simulink model "SalientPolePMSM"  (R2020b)
settings: Solver=VariableStepAuto  StartTime=0  StopTime=1  MaxStep=1e-4  RelTol=1e-4
values from neighbouring files (symbols this model uses):
  Bgain = 1    [DataSalientPolePMSM-DESKTOP-IINSHMA.m]    (also in DataSalientPolePMSM.m)
  Gcc_1ord = 1/(s/bandwidth(Gcc) + 1)    [DataSalientPolePMSM-DESKTOP-IINSHMA.m]    (also in DataSalientPolePMSM.m)
  lamdVec = mot.Ld*idVec+mot.lammg    [DataSalientPolePMSM-DESKTOP-IINSHMA.m]    (also in DataSalientPolePMSM.m)
  lamqVec = mot.Lq*iqVec    [DataSalientPolePMSM-DESKTOP-IINSHMA.m]    (also in DataSalientPolePMSM.m)
  TAB0_abc = Tabc_AB0^-1    [DataSalientPolePMSM-DESKTOP-IINSHMA.m]    (also in DataSalientPolePMSM.m)
  Tabc_AB0 = 2/3.*[     1       -1/2       -1/2 ... (first row only)    [DataSalientPolePMSM-DESKTOP-IINSHMA.m]    (also in DataSalientPolePMSM.m)
  Talphabeta_abc = Tabc_alphabeta^(-1)    [DataSalientPolePMSM-DESKTOP-IINSHMA.m]    (also in DataSalientPolePMSM.m)
undefined symbols (not defined in the file or in its folder): DiscIntNeverNeededParam, dqpll, inv, kid, kpd, magnitude, meas, mot, Obs, PI, stconv
libraries: simulink x53, pid_lib x3, powerlib x2, eeBldcCommutationLogic x1, electricdrivelib x1
(part 5 of 7)

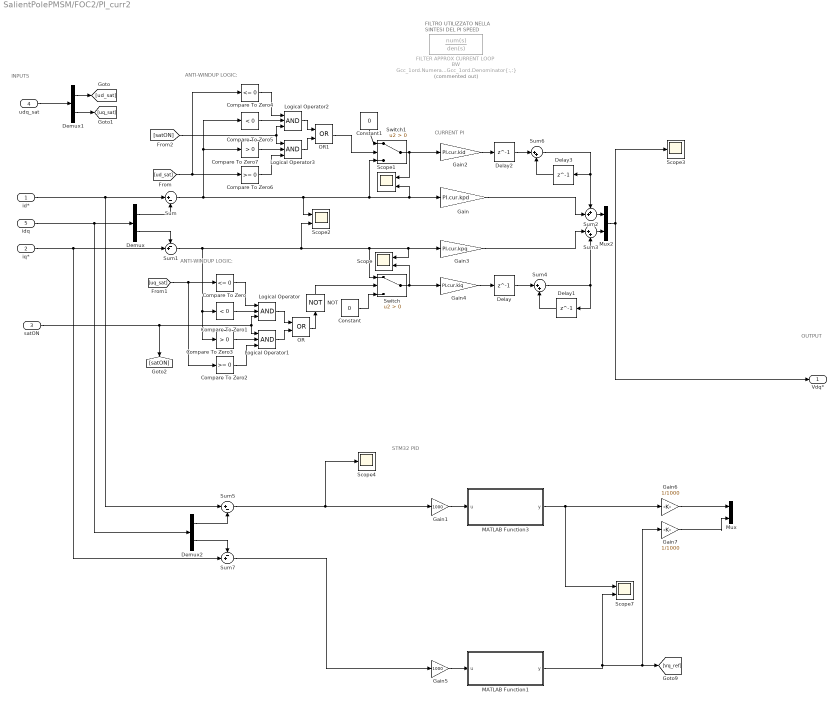
== system SalientPolePMSM/FOC2/PI_curr2 ==
  note: INPUTS
  note: OUTPUT
  note: ANTI-WINDUP LOGIC:
  note: ANTI-WINDUP LOGIC:
  note: STM32 PID
  note: FILTRO UTILIZZATO
      | NELLA SINTESI DEL
      | PI SPEED
  note: CURRENT PI
  id* : Inport
  iq* : Inport  Port=2
  satON : Inport  Port=3
  udq_sat : Inport  Port=4
  idq : Inport  Port=5
  Compare To Zero : simulink/Logic and Bit Operations/Compare To Zero  relop=<=  OutDataTypeStr=boolean  ZeroCross=off
  Compare To Zero1 : simulink/Logic and Bit Operations/Compare To Zero  relop=<  OutDataTypeStr=boolean  ZeroCross=off
  Compare To Zero2 : simulink/Logic and Bit Operations/Compare To Zero  relop=>=  OutDataTypeStr=boolean  ZeroCross=off
  Compare To Zero3 : simulink/Logic and Bit Operations/Compare To Zero  relop=>  OutDataTypeStr=boolean  ZeroCross=off
  Compare To Zero4 : simulink/Logic and Bit Operations/Compare To Zero  relop=<=  OutDataTypeStr=boolean  ZeroCross=off
  Compare To Zero5 : simulink/Logic and Bit Operations/Compare To Zero  relop=<  OutDataTypeStr=boolean  ZeroCross=off
  Compare To Zero6 : simulink/Logic and Bit Operations/Compare To Zero  relop=>=  OutDataTypeStr=boolean  ZeroCross=off
  Compare To Zero7 : simulink/Logic and Bit Operations/Compare To Zero  relop=>  OutDataTypeStr=boolean  ZeroCross=off
  Constant : Constant  Value=0
  Constant1 : Constant  Value=0
  Delay{,1..3} (4 alike) : Delay  DelayLength=1  SampleTime=PI.cur.Ts
  Demux : Demux  Outputs=2
  Demux1 : Demux  Outputs=2
  Demux2 : Demux  Outputs=2
  FILTER APPROX CURRENT LOOP BW : TransferFcn  Commented=on  Numerator=Gcc_1ord.Numerator{:,:}  Denominator=Gcc_1ord.Denominator{:,:}
  Gain : Gain  Gain=PI.cur.kpd
  Gain1 : Gain  Gain=1000
  Gain2 : Gain  Gain=PI.cur.kid
  Gain3 : Gain  Gain=PI.cur.kpq
  Gain4 : Gain  Gain=PI.cur.kiq
  Gain5 : Gain  Gain=1000
  Gain6 : Gain  Gain=1/1000
  Gain7 : Gain  Gain=1/1000
  Logical Operator{,1..3} (4 alike) : Logic  Inputs=3  AllPortsSameDT=off  OutDataTypeStr=boolean
  MATLAB Function1 : MATLAB Function  TreatAsAtomicUnit=on
  MATLAB Function3 : MATLAB Function  TreatAsAtomicUnit=on
  Mux : Mux  Inputs=2
  Mux2 : Mux  Inputs=2
  NOT : Logic  Operator=NOT  AllPortsSameDT=off  OutDataTypeStr=boolean
  OR : Logic  Operator=OR  AllPortsSameDT=off  OutDataTypeStr=boolean
  OR1 : Logic  Operator=OR  AllPortsSameDT=off  OutDataTypeStr=boolean
  Scope{,1..2,7} (4 alike) : Scope  NumInputPorts=2
  Scope3 : Scope
  Scope4 : Scope
  Sum : Sum  Inputs=|+-
  Sum1 : Sum  Inputs=-+|
  Sum2 : Sum  Inputs=++|
  Sum3 : Sum  Inputs=|++
  Sum4 : Sum  Inputs=|++
  Sum5 : Sum  Inputs=|+-
  Sum6 : Sum  Inputs=|++
  Sum7 : Sum  Inputs=-+|
  Switch : Switch  Criteria=u2 > Threshold
  Switch1 : Switch  Criteria=u2 > Threshold
  Vdq* : Outport
  wires:
  Sum/1 -> Compare To Zero5/1, Compare To Zero7/1, Switch1/3, Gain/1, Scope1/2, Scope2/1
  Switch/1 -> Gain4/1, Scope/2
  MATLAB Function1/1(y) -> Scope7/2, Gain7/1, [Vq_ref]
  MATLAB Function3/1(y) -> Scope7/1, Gain6/1
  Demux/2 -> Sum1/1
  Gain2/1 -> Delay2/1
  Sum6/1 -> Sum2/1, Delay3/1
  Delay2/1 -> Sum6/1
  Delay3/1 -> Sum6/2
  Delay1/1 -> Sum4/2
  Delay/1 -> Sum4/1
  iq*/1 -> Sum7/2, Sum1/2
  Demux1/2 -> [uq_sat]
  Demux1/1 -> [ud_sat]
  udq_sat/1 -> Demux1/1
  Switch1/1 -> Gain2/1, Scope1/1
  Constant1/1 -> Switch1/1
  OR1/1 -> Switch1/2
  [satON] -> Logical Operator3/1, Logical Operator2/3
  Logical Operator2/1 -> OR1/1
  Logical Operator3/1 -> OR1/2
  Compare To Zero5/1 -> Logical Operator2/2
  Compare To Zero4/1 -> Logical Operator2/1
  Compare To Zero6/1 -> Logical Operator3/3
  [ud_sat] -> Compare To Zero6/1, Compare To Zero4/1
  Compare To Zero7/1 -> Logical Operator3/2
  Compare To Zero3/1 -> Logical Operator1/2
  [uq_sat] -> Compare To Zero/1, Compare To Zero2/1
  Compare To Zero2/1 -> Logical Operator1/3
  Compare To Zero/1 -> Logical Operator/1
  Compare To Zero1/1 -> Logical Operator/2
  Logical Operator1/1 -> OR/2
  Logical Operator/1 -> OR/1
  NOT/1 -> Switch/2
  OR/1 -> NOT/1
  Constant/1 -> Switch/3
  Gain3/1 -> Sum3/1
  Gain4/1 -> Delay/1
  Gain/1 -> Sum2/2
  Sum1/1 -> Compare To Zero1/1, Compare To Zero3/1, Gain3/1, Scope/1, Switch/1, Scope2/2
  Sum4/1 -> Sum3/2, Delay1/1
  Sum2/1 -> Mux2/1
  Sum3/1 -> Mux2/2
  Demux/1 -> Sum/2
  idq/1 -> Demux2/1, Demux/1
  satON/1 -> Logical Operator1/1, Logical Operator/3, [satON]
  Demux2/2 -> Sum7/1
  Demux2/1 -> Sum5/2
  Sum5/1 -> Scope4/1, Gain1/1
  Sum7/1 -> Gain5/1
  id*/1 -> Sum5/1, Sum/1
  Mux2/1 -> Vdq*/1, Scope3/1
  Gain1/1 -> MATLAB Function3/1(u)
  Gain5/1 -> MATLAB Function1/1(u)
  Gain6/1 -> Mux/1
  Gain7/1 -> Mux/2

== system SalientPolePMSM/FOC2/Rev_Park ==
  note: OUTPUT
  note: INPUTS
  dq : Inport
  thme : Inport  Port=2
  Add2 : Sum  Inputs=+-
  Add3 : Sum
  Cos2 : Trigonometry  Operator=cos
  Demux2 : Demux  Outputs=2
  Mux1 : Mux  Inputs=2
  Product{,1..3} (4 alike) : Product
  Sin2 : Trigonometry
  AB : Outport
  wires:
  Mux1/1 -> AB/1
  Sin2/1 -> Product1/2, Product2/2
  Demux2/2 -> Product1/1, Product3/2
  Product2/1 -> Add3/1
  Product3/1 -> Add3/2
  thme/1 -> Sin2/1, Cos2/1
  Demux2/1 -> Product2/1, Product/1
  Cos2/1 -> Product3/1, Product/2
  Product1/1 -> Add2/2
  Add3/1 -> Mux1/2
  Add2/1 -> Mux1/1
  Product/1 -> Add2/1
  dq/1 -> Demux2/1

== system SalientPolePMSM/FOC2/Rev_Park 2 ==
  note: OUTPUT
  note: INPUTS
  dq : Inport
  thme : Inport  Port=2
  Add2 : Sum
  Add3 : Sum  Inputs=+-
  Cos2 : Trigonometry  Operator=cos
  Demux2 : Demux  Outputs=2
  Gain2 : Gain  Gain=2
  Gain3 : Gain  Gain=-1/sqrt(3)
  Mux1 : Mux  Inputs=2
  Product{,1..3,5} (5 alike) : Product
  Sin2 : Trigonometry
  AB : Outport
  wires:
  Product3/1 -> Add2/1
  Demux2/2 -> Product2/1, Product3/2
  Mux1/1 -> AB/1
  Sin2/1 -> Product1/2, Product2/2
  thme/1 -> Sin2/1, Cos2/1
  Cos2/1 -> Product/2, Product3/1
  Product1/1 -> Add2/2
  dq/1 -> Demux2/1
  ? -> Gain2/1
  Product5/1 -> Gain3/1
  Gain2/1 -> Product5/2
  ? -> Product5/1
  Gain3/1 -> ?
  Add3/1 -> Mux1/2
  Add2/1 -> Mux1/1
  Product2/1 -> Add3/2
  Product/1 -> Add3/1
  Demux2/1 -> Product/1, Product1/1

== system SalientPolePMSM/FOC2/Subsystem1 ==
  note: OUTPUT
  note: INPUTS
  dq : Inport
  Demux2 : Demux  Outputs=2
  Gain : Gain  Gain=-1
  Mux1 : Mux  Inputs=2
  qd : Outport
  wires:
  Mux1/1 -> qd/1
  dq/1 -> Demux2/1
  Demux2/1 -> Mux1/2
  Demux2/2 -> Gain/1
  Gain/1 -> Mux1/1

== system SalientPolePMSM/FOC2/Subsystem4 ==
  note: OUTPUT
  note: INPUTS
  dq : Inport
  thme : Inport  Port=2
  Add2 : Sum  Inputs=+-
  Add3 : Sum
  Cos2 : Trigonometry  Operator=cos
  Demux2 : Demux  Outputs=2
  Mux1 : Mux  Inputs=2
  Product{,1..3} (4 alike) : Product
  Sin2 : Trigonometry
  AB : Outport
  wires:
  Mux1/1 -> AB/1
  Sin2/1 -> Product1/2, Product2/2
  Demux2/2 -> Product1/1, Product3/2
  Product2/1 -> Add3/1
  Product3/1 -> Add3/2
  thme/1 -> Sin2/1, Cos2/1
  Demux2/1 -> Product2/1, Product/1
  Cos2/1 -> Product3/1, Product/2
  Product1/1 -> Add2/2
  Add3/1 -> Mux1/2
  Add2/1 -> Mux1/1
  Product/1 -> Add2/1
  dq/1 -> Demux2/1

== system SalientPolePMSM/Feedback1/Hall Decoder2 ==
  thm : Inport
  wm : Inport  Port=2
  Delay1 : Delay  DelayLength=1
  Demux : Demux
  Discrete-Time Integrator : DiscreteIntegrator  SampleTime=1/1000  ICPrevOutput=DiscIntNeverNeededParam  ICPrevScaledInput=DiscIntNeverNeededParam
  Gain : Gain  Gain=mot.p
  Gain1 : Gain  Gain=mot.p
  Lookup table hall sensor : MATLAB Function  TreatAsAtomicUnit=on  SystemSampleTime=meas.hall.Ts
  Scope : Scope  NumInputPorts=3
  Scope1 : Scope  NumInputPorts=3
  Terminator : Terminator
  Terminator1 : Terminator
  Terminator2 : Terminator
  Update speed and angle : MATLAB Function  TreatAsAtomicUnit=on
  wires:
  wm/1 -> Gain/1
  Lookup table hall sensor/1(Hall) -> Scope/3, Demux/1
  thm/1 -> Gain1/1
  Gain1/1 -> Scope/1, Lookup table hall sensor/1(thme)
  Demux/3 -> Update speed and angle/1(Hall_state), Delay1/1, Terminator1/1
  Demux/2 -> Terminator/1
  Demux/1 -> Terminator2/1
  Delay1/1 -> Scope1/1, Update speed and angle/2(prev_Hall_state)
  Update speed and angle/1(thme) -> Scope/2
  Discrete-Time Integrator/1 -> Update speed and angle/3(prev_wme)
  Gain/1 -> Discrete-Time Integrator/1  "wme"

== system SalientPolePMSM/Feedback1/Rev_Park + Rev_Clarke2 ==
  note: INPUTS
  Iabc : Inport
  thme1 : Inport  Port=2
  Add1 : Sum  Inputs=+-
  Add4 : Sum
  Cos1 : Trigonometry  Operator=cos
  Demux1 : Demux  Outputs=3
  Gain : Gain  Gain=sqrt(3)
  Gain1 : Gain  Gain=1/2
  Mux : Mux  Inputs=2
  Product{4..7} (4 alike) : Product
  Sin1 : Trigonometry
  Sum2 : Sum  Inputs=--|
  Terminator : Terminator
  dq : Outport
  wires:
  Demux1/3 -> Terminator/1
  Cos1/1 -> Product6/2, Product7/1
  Product5/1 -> Add1/2
  Sin1/1 -> Product5/2, Product4/2
  Product6/1 -> Add4/1
  Product4/1 -> Add4/2
  Product7/1 -> Add1/1
  Gain/1 -> Sum2/2
  Sum2/1 -> Gain1/1
  Gain1/1 -> Product7/2, Product4/1
  Demux1/1 -> Product5/1, Product6/1, Sum2/1
  Mux/1 -> dq/1
  Add1/1 -> Mux/1
  Add4/1 -> Mux/2
  Iabc/1 -> Demux1/1
  Demux1/2 -> Gain/1
  thme1/1 -> Sin1/1, Cos1/1

== system SalientPolePMSM/Feedback2/Hall Decoder2 ==
  thm : Inport
  wm : Inport  Port=2
  Delay1 : Delay  DelayLength=1
  Demux : Demux
  Discrete-Time Integrator : DiscreteIntegrator  SampleTime=1/1000  ICPrevOutput=DiscIntNeverNeededParam  ICPrevScaledInput=DiscIntNeverNeededParam
  Gain : Gain  Gain=mot.p
  Gain1 : Gain  Gain=mot.p
  Lookup table hall sensor : MATLAB Function  TreatAsAtomicUnit=on  SystemSampleTime=meas.hall.Ts
  Scope1 : Scope  NumInputPorts=3
  Terminator : Terminator
  Terminator1 : Terminator
  Terminator2 : Terminator
  Update speed and angle : MATLAB Function  TreatAsAtomicUnit=on
  wires:
  wm/1 -> Gain/1
  Lookup table hall sensor/1(Hall) -> Demux/1
  thm/1 -> Gain1/1
  Gain1/1 -> Lookup table hall sensor/1(thme)
  Demux/3 -> Update speed and angle/1(Hall_state), Delay1/1, Terminator1/1
  Demux/2 -> Terminator/1
  Demux/1 -> Terminator2/1
  Delay1/1 -> Scope1/1, Update speed and angle/2(prev_Hall_state)
  Discrete-Time Integrator/1 -> Update speed and angle/3(prev_wme)
  Gain/1 -> Discrete-Time Integrator/1  "wme"

== system SalientPolePMSM/Feedback2/Rev_Park + Rev_Clarke2 ==
  note: INPUTS
  Iabc : Inport
  thme1 : Inport  Port=2
  Add1 : Sum  Inputs=+-
  Add4 : Sum
  Cos1 : Trigonometry  Operator=cos
  Demux1 : Demux  Outputs=3
  Gain : Gain  Gain=sqrt(3)
  Gain1 : Gain  Gain=1/2
  Mux : Mux  Inputs=2
  Product{4..7} (4 alike) : Product
  Sin1 : Trigonometry
  Sum2 : Sum  Inputs=--|
  Terminator : Terminator
  dq : Outport
  wires:
  Demux1/3 -> Terminator/1
  Cos1/1 -> Product6/2, Product7/1
  Product5/1 -> Add1/2
  Sin1/1 -> Product5/2, Product4/2
  Product6/1 -> Add4/1
  Product4/1 -> Add4/2
  Product7/1 -> Add1/1
  Gain/1 -> Sum2/2
  Sum2/1 -> Gain1/1
  Gain1/1 -> Product7/2, Product4/1
  Demux1/1 -> Product5/1, Product6/1, Sum2/1
  Mux/1 -> dq/1
  Add1/1 -> Mux/1
  Add4/1 -> Mux/2
  Iabc/1 -> Demux1/1
  Demux1/2 -> Gain/1
  thme1/1 -> Sin1/1, Cos1/1

== system SalientPolePMSM/INVERTER/INVERTER power driver ==
  note: solo Tpwm/2 perchè
      | controllo tempo discreto
  note: OUTPUTS:
  note: INPUTS:
  note: INVERTER:
      | (-Ubus/2  :  +Ubus/2)
  duties : Inport
  uBus : Inport  Port=2
  iabc : Inport  Port=3
  Constant1 : Constant  Value=0.5
  Inverter non idealities : Subsystem
  Product : Product
  Subtract : Sum  Inputs=+-
  Transport Delay : TransportDelay  DelayTime=inv.Tpwm/2
  delay_aproximation : Subsystem  Commented=on
  uabc_n* : Outport
  uabc_n*nonideal : Outport  Port=2
  wires:
  Transport Delay/1 -> uabc_n*/1
  Subtract/1 -> Product/1
  Product/1 -> Transport Delay/1, Inverter non idealities/1(uabc)  "uabc"
  uBus/1 -> Product/2, Inverter non idealities/2(uBus)
  Constant1/1 -> Subtract/2
  Inverter non idealities/1(uabc_dist) -> uabc_n*nonideal/1
  duties/1 -> Subtract/1
  iabc/1 -> Inverter non idealities/3(iabc)

== system SalientPolePMSM/INVERTER/SVM algorithm ==
  note: OUTPUT
  note: Decide whether
      | to use circle or
      | hexagonal saturation
  note: INPUTS:
      | voltage references
      | Alpha Beta axes
  UABref : Inport  PortDimensions=2
  uBus : Inport  Port=2  PortDimensions=1
  MATLAB Function : MATLAB Function  TreatAsAtomicUnit=on
  MATLAB Function1 : MATLAB Function  TreatAsAtomicUnit=on
  MATLAB Function2 : MATLAB Function  TreatAsAtomicUnit=on
  MATLAB Function3 : MATLAB Function  TreatAsAtomicUnit=on
  Manual Switch : ManualSwitch  CurrentSetting=0
  OR : Logic  Operator=OR  IconShape=distinctive  AllPortsSameDT=off  OutDataTypeStr=boolean
  Scope : Scope
  XY Graph : simulink/Sinks/XY Graph  xmin=-350  xmax=350  ymin=-350  ymax=350  st=-1
  duties : Outport  PortDimensions=3
  satON : Outport  Port=2  PortDimensions=1
  wires:
  MATLAB Function3/1(uAref_sat) -> XY Graph/1  "uAref_sat"
  MATLAB Function3/2(uBref_sat) -> XY Graph/2  "uBref_sat"
  MATLAB Function/1(sector) -> MATLAB Function3/1(sid), MATLAB Function2/1(sid)
  [UBUS] -> MATLAB Function2/3(uBus)
  UABref/1 -> MATLAB Function1/1(UABref), Manual Switch/1, MATLAB Function/1(uABref)
  [UBUS] -> MATLAB Function1/2(uBus)
  MATLAB Function1/1(uABref_sat) -> Manual Switch/2
  Manual Switch/1 -> MATLAB Function3/3(uABref), MATLAB Function2/2(uABref)
  uBus/1 -> [UBUS]
  MATLAB Function3/3(duties) -> duties/1
  MATLAB Function3/4(satON) -> OR/1
  MATLAB Function1/2(satON) -> OR/2
  OR/1 -> satON/1
  MATLAB Function2/1(Tm_m1_0) -> Scope/1, MATLAB Function3/2(Tm_m1_0)

== system SalientPolePMSM/SENSORLESS ALGORITHM/DECOUPLING ==
  note: OUTPUTS:
  note: INPUTS:
  idq_est : Inport
  udq_est : Inport  Port=2
  wme_est : Inport  Port=3
  Demux1 : Demux  Outputs=2
  Demux2 : Demux  Outputs=2
  Gain10 : Gain  Gain=dqpll.Lq
  Gain11 : Gain  Gain=dqpll.Lq
  Mux : Mux  Inputs=2
  Mux1 : Mux  Inputs=2
  Product : Product
  Product1 : Product
  Sum1 : Sum  Inputs=-+|
  Sum3 : Sum  Inputs=++|
  ud' id : Outport
  uq' iq : Outport  Port=2
  wires:
  Sum1/1 -> Mux1/1
  Product/1 -> Gain10/1
  Product1/1 -> Gain11/1
  Gain10/1 -> Sum3/1
  Gain11/1 -> Sum1/1
  Sum3/1 -> Mux/1
  idq_est/1 -> Demux2/1
  udq_est/1 -> Demux1/1
  Mux1/1 -> uq' iq/1
  Mux/1 -> ud' id/1
  wme_est/1 -> [WME_EST]
  [WME_EST] -> Product1/2
  [WME_EST] -> Product/1
  Demux2/2 -> [IQ]
  [IQ] -> Product/2
  [IQ] -> Mux1/2
  Demux2/1 -> [ID]
  [ID] -> Mux/2
  [ID] -> Product1/1
  Demux1/1 -> [UD]
  Demux1/2 -> [UQ]
  [UD] -> Sum3/2
  [UQ] -> Sum1/2

== system SalientPolePMSM/SENSORLESS ALGORITHM/ESTIMETOR ed ==
  ud : Inport
  id : Inport  Port=2
  Gain : Gain  Gain=dqpll.est.g*dqpll.Ld - dqpll.R
  Gain1 : Gain  Gain=dqpll.est.g*dqpll.Ld
  Sum : Sum  Inputs=|+-
  Sum1 : Sum  Inputs=+|+
  Transfer Fcn : TransferFcn  Numerator=[dqpll.est.g]  Denominator=[1 dqpll.est.g]
  ed : Outport
  wires:
  Gain1/1 -> Sum/2
  Sum/1 -> ed/1
  Transfer Fcn/1 -> Sum/1
  id/1 -> Gain1/1, Gain/1
  Gain/1 -> Sum1/2
  Sum1/1 -> Transfer Fcn/1
  ud/1 -> Sum1/1

== system SalientPolePMSM/SENSORLESS ALGORITHM/ESTIMETOR eq ==
  uq : Inport
  iq : Inport  Port=2
  Gain : Gain  Gain=dqpll.est.g*dqpll.Ld - dqpll.R
  Gain1 : Gain  Gain=dqpll.est.g*dqpll.Ld
  Sum : Sum  Inputs=|+-
  Sum1 : Sum  Inputs=+|+
  Transfer Fcn : TransferFcn  Numerator=[dqpll.est.g]  Denominator=[1 dqpll.est.g]
  eq : Outport
  wires:
  uq/1 -> Sum1/1
  Sum1/1 -> Transfer Fcn/1
  Gain/1 -> Sum1/2
  iq/1 -> Gain/1, Gain1/1
  Transfer Fcn/1 -> Sum/1
  Sum/1 -> eq/1
  Gain1/1 -> Sum/2

== system SalientPolePMSM/SENSORLESS ALGORITHM/PI ==
  e : Inport
  Gain6 : Gain  Gain=dqpll.PI.ki
  Gain7 : Gain  Gain=dqpll.PI.kp
  Integrator : Integrator
  Sum2 : Sum  Inputs=++|
  w_est : Outport
  wires:
  Gain7/1 -> Sum2/2
  Sum2/1 -> w_est/1  "w_est"
  e/1 -> Integrator/1, Gain7/1
  Integrator/1 -> Gain6/1
  Gain6/1 -> Sum2/1

== system SalientPolePMSM/SENSORLESS ALGORITHM/PII ==
  e : Inport
  Add : Sum  Inputs=+++
  Gain1 : Gain  Gain=dqpll.PI.k3
  Gain6 : Gain  Gain=dqpll.PI.k2
  Gain7 : Gain  Gain=dqpll.PI.k1
  Integrator : Integrator
  Integrator1 : Integrator
  Integrator2 : Integrator
  w_est : Outport
  wires:
  Gain6/1 -> Add/1
  Integrator/1 -> Gain6/1
  e/1 -> Integrator1/1, Gain7/1, Integrator/1
  Add/1 -> w_est/1  "w_est"
  Gain7/1 -> Add/2
  Integrator1/1 -> Integrator2/1
  Gain1/1 -> Add/3
  Integrator2/1 -> Gain1/1

== system SalientPolePMSM/SENSORLESS ALGORITHM/Subsystem1 ==
  note: OUTPUT
  note: INPUTS
  abc : Inport
  thme : Inport  Port=2
  Add2 : Sum
  Add3 : Sum  Inputs=-+
  Cos2 : Trigonometry  Operator=cos
  Demux2 : Demux  Outputs=3
  Gain : Gain  Gain=Tabc_AB0  Multiplication=Matrix(K*u) (u vector)
  Mux1 : Mux  Inputs=2
  Product{,1..3} (4 alike) : Product
  Sin2 : Trigonometry
  Terminator : Terminator
  dq : Outport
  wires:
  Mux1/1 -> dq/1
  Sin2/1 -> Product1/2, Product2/2
  Demux2/2 -> Product3/2, Product1/1
  Product2/1 -> Add3/1
  Product3/1 -> Add3/2
  thme/1 -> Sin2/1, Cos2/1
  Demux2/1 -> Product2/1, Product/1
  Cos2/1 -> Product3/1, Product/2
  Product1/1 -> Add2/2
  Add3/1 -> Mux1/2
  Add2/1 -> Mux1/1
  Product/1 -> Add2/1
  Gain/1 -> Demux2/1  "AB0"
  Demux2/3 -> Terminator/1
  abc/1 -> Gain/1

== system SalientPolePMSM/SENSORLESS ALGORITHM/Subsystem2 ==
  note: INPUTS
  note: OUTPUT
  abc : Inport
  thme : Inport  Port=2
  Add2 : Sum
  Add3 : Sum  Inputs=-+
  Cos2 : Trigonometry  Operator=cos
  Demux2 : Demux  Outputs=3
  Gain : Gain  Gain=Tabc_AB0  Multiplication=Matrix(K*u) (u vector)
  Mux1 : Mux  Inputs=2
  Product{,1..3} (4 alike) : Product
  Sin2 : Trigonometry
  Terminator : Terminator
  dq : Outport
  wires:
  abc/1 -> Gain/1
  Demux2/3 -> Terminator/1
  Gain/1 -> Demux2/1  "AB0"
  Product/1 -> Add2/1
  Add2/1 -> Mux1/1
  Add3/1 -> Mux1/2
  Product1/1 -> Add2/2
  Cos2/1 -> Product/2, Product3/1
  Demux2/1 -> Product/1, Product2/1
  thme/1 -> Cos2/1, Sin2/1
  Product3/1 -> Add3/2
  Product2/1 -> Add3/1
  Demux2/2 -> Product1/1, Product3/2
  Sin2/1 -> Product2/2, Product1/2
  Mux1/1 -> dq/1

== system SalientPolePMSM/SENSORLESS ALGORITHM1/DECOUPLING ==
  note: OUTPUTS:
  note: INPUTS:
  idq_est : Inport
  udq_est : Inport  Port=2
  wme_est : Inport  Port=3
  Demux1 : Demux  Outputs=2
  Demux2 : Demux  Outputs=2
  Gain10 : Gain  Gain=dqpll.Lq
  Gain11 : Gain  Gain=dqpll.Lq
  Mux : Mux  Inputs=2
  Mux1 : Mux  Inputs=2
  Product : Product
  Product1 : Product
  Sum1 : Sum  Inputs=-+|
  Sum3 : Sum  Inputs=++|
  ud' id : Outport
  uq' iq : Outport  Port=2
  wires:
  Sum1/1 -> Mux1/1
  Product/1 -> Gain10/1
  Product1/1 -> Gain11/1
  Gain10/1 -> Sum3/1
  Gain11/1 -> Sum1/1
  Sum3/1 -> Mux/1
  idq_est/1 -> Demux2/1
  udq_est/1 -> Demux1/1
  Mux1/1 -> uq' iq/1
  Mux/1 -> ud' id/1
  wme_est/1 -> [WME_EST]
  [WME_EST] -> Product1/2
  [WME_EST] -> Product/1
  Demux2/2 -> [IQ]
  [IQ] -> Product/2
  [IQ] -> Mux1/2
  Demux2/1 -> [ID]
  [ID] -> Mux/2
  [ID] -> Product1/1
  Demux1/1 -> [UD]
  Demux1/2 -> [UQ]
  [UD] -> Sum3/2
  [UQ] -> Sum1/2

== system SalientPolePMSM/SENSORLESS ALGORITHM1/ESTIMETOR ed ==
  ud : Inport
  id : Inport  Port=2
  Gain : Gain  Gain=dqpll.est.g*dqpll.Ld - dqpll.R
  Gain1 : Gain  Gain=dqpll.est.g*dqpll.Ld
  Sum : Sum  Inputs=|+-
  Sum1 : Sum  Inputs=+|+
  Transfer Fcn : TransferFcn  Numerator=[dqpll.est.g]  Denominator=[1 dqpll.est.g]
  ed : Outport
  wires:
  Gain1/1 -> Sum/2
  Sum/1 -> ed/1
  Transfer Fcn/1 -> Sum/1
  id/1 -> Gain1/1, Gain/1
  Gain/1 -> Sum1/2
  Sum1/1 -> Transfer Fcn/1
  ud/1 -> Sum1/1

== system SalientPolePMSM/SENSORLESS ALGORITHM1/ESTIMETOR eq ==
  uq : Inport
  iq : Inport  Port=2
  Gain : Gain  Gain=dqpll.est.g*dqpll.Ld - dqpll.R
  Gain1 : Gain  Gain=dqpll.est.g*dqpll.Ld
  Sum : Sum  Inputs=|+-
  Sum1 : Sum  Inputs=+|+
  Transfer Fcn : TransferFcn  Numerator=[dqpll.est.g]  Denominator=[1 dqpll.est.g]
  eq : Outport
  wires:
  uq/1 -> Sum1/1
  Sum1/1 -> Transfer Fcn/1
  Gain/1 -> Sum1/2
  iq/1 -> Gain/1, Gain1/1
  Transfer Fcn/1 -> Sum/1
  Sum/1 -> eq/1
  Gain1/1 -> Sum/2

== system SalientPolePMSM/SENSORLESS ALGORITHM1/PI ==
  e : Inport
  Gain6 : Gain  Gain=dqpll.PI.ki
  Gain7 : Gain  Gain=dqpll.PI.kp
  Integrator : Integrator
  Sum2 : Sum  Inputs=++|
  w_est : Outport
  wires:
  Gain7/1 -> Sum2/2
  Sum2/1 -> w_est/1  "w_est"
  e/1 -> Integrator/1, Gain7/1
  Integrator/1 -> Gain6/1
  Gain6/1 -> Sum2/1

== system SalientPolePMSM/SENSORLESS ALGORITHM1/PII ==
  e : Inport
  Add : Sum  Inputs=+++
  Gain1 : Gain  Gain=dqpll.PI.k3
  Gain6 : Gain  Gain=dqpll.PI.k2
  Gain7 : Gain  Gain=dqpll.PI.k1
  Integrator : Integrator
  Integrator1 : Integrator
  Integrator2 : Integrator
  w_est : Outport
  wires:
  Gain6/1 -> Add/1
  Integrator/1 -> Gain6/1
  e/1 -> Integrator1/1, Gain7/1, Integrator/1
  Add/1 -> w_est/1  "w_est"
  Gain7/1 -> Add/2
  Integrator1/1 -> Integrator2/1
  Gain1/1 -> Add/3
  Integrator2/1 -> Gain1/1

== system SalientPolePMSM/SENSORLESS ALGORITHM1/Subsystem1 ==
  note: OUTPUT
  note: INPUTS
  abc : Inport
  thme : Inport  Port=2
  Add2 : Sum
  Add3 : Sum  Inputs=-+
  Cos2 : Trigonometry  Operator=cos
  Demux2 : Demux  Outputs=3
  Gain : Gain  Gain=Tabc_AB0  Multiplication=Matrix(K*u) (u vector)
  Mux1 : Mux  Inputs=2
  Product{,1..3} (4 alike) : Product
  Sin2 : Trigonometry
  Terminator : Terminator
  dq : Outport
  wires:
  Mux1/1 -> dq/1
  Sin2/1 -> Product1/2, Product2/2
  Demux2/2 -> Product3/2, Product1/1
  Product2/1 -> Add3/1
  Product3/1 -> Add3/2
  thme/1 -> Sin2/1, Cos2/1
  Demux2/1 -> Product2/1, Product/1
  Cos2/1 -> Product3/1, Product/2
  Product1/1 -> Add2/2
  Add3/1 -> Mux1/2
  Add2/1 -> Mux1/1
  Product/1 -> Add2/1
  Gain/1 -> Demux2/1  "AB0"
  Demux2/3 -> Terminator/1
  abc/1 -> Gain/1

== system SalientPolePMSM/SENSORLESS ALGORITHM1/Subsystem2 ==
  note: INPUTS
  note: OUTPUT
  abc : Inport
  thme : Inport  Port=2
  Add2 : Sum
  Add3 : Sum  Inputs=-+
  Cos2 : Trigonometry  Operator=cos
  Demux2 : Demux  Outputs=3
  Gain : Gain  Gain=Tabc_AB0  Multiplication=Matrix(K*u) (u vector)
  Mux1 : Mux  Inputs=2
  Product{,1..3} (4 alike) : Product
  Sin2 : Trigonometry
  Terminator : Terminator
  dq : Outport
  wires:
  abc/1 -> Gain/1
  Demux2/3 -> Terminator/1
  Gain/1 -> Demux2/1  "AB0"
  Product/1 -> Add2/1
  Add2/1 -> Mux1/1
  Add3/1 -> Mux1/2
  Product1/1 -> Add2/2
  Cos2/1 -> Product/2, Product3/1
  Demux2/1 -> Product/1, Product2/1
  thme/1 -> Cos2/1, Sin2/1
  Product3/1 -> Add3/2
  Product2/1 -> Add3/1
  Demux2/2 -> Product1/1, Product3/2
  Sin2/1 -> Product2/2, Product1/2
  Mux1/1 -> dq/1

== system SalientPolePMSM/Synchronous motor1/Clarke + Park 1 ==
  note: INPUTS
  note: OUTPUT
  abc : Inport
  thme : Inport  Port=2
  Add2 : Sum
  Add3 : Sum  Inputs=-+
  Cos2 : Trigonometry  Operator=cos
  Demux1 : Demux  Outputs=3
  Demux2 : Demux  Outputs=3
  Gain1 : Gain  Gain=Tabc_AB0  Multiplication=Matrix(K*u) (u vector)
  Gain10 : Gain  Gain=-1/sqrt(3)
  Gain9 : Gain  Gain=2
  Mux1 : Mux  Inputs=2
  Mux2 : Mux  Inputs=3
  Product{,1..3} (4 alike) : Product
  Scope : Scope  NumInputPorts=2
  Sin2 : Trigonometry
  Sum5 : Sum  Inputs=++|
  Terminator : Terminator
  dq : Outport
  wires:
  Demux2/3 -> Terminator/1
  Product/1 -> Add2/1
  Product1/1 -> Add2/2
  Cos2/1 -> Product/2, Product3/1
  Demux2/1 -> Product3/2, Product1/1
  thme/1 -> Cos2/1, Sin2/1
  Product3/1 -> Add3/2
  Product2/1 -> Add3/1
  Demux2/2 -> Product2/1, Product/1
  Sin2/1 -> Product2/2, Product1/2
  Mux1/1 -> dq/1
  Add3/1 -> Mux1/2
  Add2/1 -> Mux1/1
  Sum5/1 -> Gain10/1
  Gain9/1 -> Sum5/2
  Demux1/2 -> Gain9/1
  Demux1/3 -> Mux2/3
  Demux1/1 -> Mux2/1, Sum5/1
  Gain10/1 -> Mux2/2
  abc/1 -> Gain1/1, Demux1/1
  Gain1/1 -> Scope/1, Demux2/1

== system SalientPolePMSM/Synchronous motor1/Rev_Park + Rev_Clarke ==
  note: INPUTS
  dq : Inport
  thme1 : Inport  Port=2
  Add1 : Sum  Inputs=+-
  Add3 : Sum  Inputs=--
  Add4 : Sum
  Cos1 : Trigonometry  Operator=cos
  Demux1 : Demux  Outputs=3
  Gain2 : Gain  Gain=2
  Gain3 : Gain  Gain=-1/sqrt(3)
  Gain4 : Gain  Gain=Talphabeta_abc  Multiplication=Matrix(K*u) (u vector)
  Mux2 : Mux  Inputs=3
  Product{4..7} (4 alike) : Product
  Scope2 : Scope  NumInputPorts=5
  Scope3 : Scope  NumInputPorts=2
  Sin1 : Trigonometry
  Sum1 : Sum  Inputs=++|
  Terminator : Terminator
  abc : Outport
  wires:
  Demux1/3 -> Terminator/1
  dq/1 -> Demux1/1
  Cos1/1 -> Product6/2, Product7/1
  Product5/1 -> Add1/2
  Sin1/1 -> Product5/2, Product4/2
  Product6/1 -> Add4/1
  thme1/1 -> Sin1/1, Cos1/1
  Product4/1 -> Add4/2
  Demux1/1 -> Product5/1, Product6/1
  Product7/1 -> Add1/1
  Demux1/2 -> Product7/2, Product4/1
  Gain3/1 -> Scope2/4, Mux2/2, Add3/2
  Sum1/1 -> Gain3/1
  Gain2/1 -> Sum1/2
  Add3/1 -> Scope2/5, Mux2/3
  Add1/1 -> Scope2/1, Scope2/3, Mux2/1, Add3/1, Sum1/1
  Add4/1 -> Scope2/2, Gain2/1
  ? -> Scope3/2
  Gain4/1 -> Scope3/1
  Mux2/1 -> abc/1

== system SalientPolePMSM/Synchronous motor1/SPM Motor ==
  note: Mechanical Part
  note: Electrical Part
  dq : Inport
  Demux : Demux  Outputs=2
  Divide : Product  Inputs=*/  RndMeth=Zero  SaturateOnIntegerOverflow=on
  Gain : Gain  Gain=mot.Ld
  Gain3 : Gain  Gain=mot.Lq
  Gain4 : Gain  Gain=mot.lammg
  Gain5 : Gain  Gain=3/2*mot.lammg*mot.p
  Gain6 : Gain  Gain=mot.p
  Integrator : Integrator
  MATLAB Function : MATLAB Function  TreatAsAtomicUnit=on
  Product : Product
  Product1 : Product
  Scope : Scope
  Scope2 : Scope
  Scope3 : Scope
  Sum : Sum  Inputs=|++
  Sum1 : Sum  Inputs=-+-
  Sum2 : Sum  Inputs=|+-
  Sum4 : Sum  Inputs=++|
  Transfer Fcn : TransferFcn  Denominator=[mot.Ld mot.R]
  Transfer Fcn1 : TransferFcn  Denominator=[mot.Lq mot.R]
  Transfer Fcn2 : TransferFcn  Denominator=[mot.J mot.B]
  theta_me : Outport
  w_me : Outport  Port=2
  wires:
  dq/1 -> Demux/1
  [TAUL] -> Sum2/2
  Sum/1 -> Transfer Fcn/1
  Gain3/1 -> Sum/2
  Gain/1 -> Sum1/1
  Integrator/1 -> Sum4/2  "theta_me"
  Sum2/1 -> Transfer Fcn2/1
  Transfer Fcn/1 -> Product/1  "id"
  Gain6/1 -> Product/2, Product1/1, Integrator/1, w_me/1, Scope3/1, Gain4/1  "w_me"
  Product/1 -> Gain/1
  Demux/2 -> Sum1/2
  Product1/1 -> Gain3/1
  Gain4/1 -> Sum1/3
  Sum1/1 -> Transfer Fcn1/1
  Sum4/1 -> theta_me/1
  Demux/1 -> Sum/1
  Transfer Fcn1/1 -> Gain5/1, Scope2/1, Product1/2  "iq"
  Transfer Fcn2/1 -> Gain6/1  "w_m"
  MATLAB Function/1(B) -> Divide/2
  Gain5/1 -> Sum2/1, Scope/1  "tau"

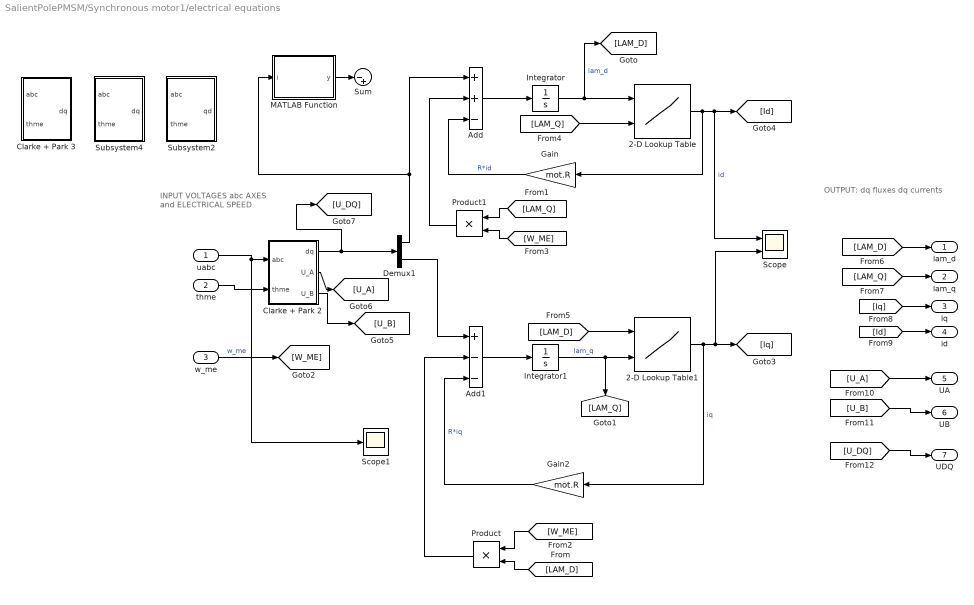
== system SalientPolePMSM/Synchronous motor1/electrical equations ==
  note: INPUT VOLTAGES
      | abc AXES and
      | ELECTRICAL
      | SPEED
  note: OUTPUT:
      | dq fluxes
      | dq currents
  uabc : Inport
  thme : Inport  Port=2
  w_me : Inport  Port=3
  2-D Lookup Table : Lookup_n-D  BreakpointsForDimension1=lamdVec  BreakpointsForDimension2=lamqVec  Table=idMap'  InternalRulePriority=Speed  RndMeth=Simplest  InputSameDT=on
      settings: InputPortMap=u0,u1
  2-D Lookup Table1 : Lookup_n-D  BreakpointsForDimension1=lamdVec  BreakpointsForDimension2=lamqVec  Table=iqMap'  InternalRulePriority=Speed  RndMeth=Simplest  InputSameDT=on
      settings: InputPortMap=u0,u1
  Add : Sum  Inputs=++-
  Add1 : Sum  Inputs=+--
  Clarke + Park 2 : Subsystem
  Clarke + Park 3 : Subsystem
  Demux1 : Demux  Outputs=2
  Gain : Gain  Gain=mot.R
  Gain2 : Gain  Gain=mot.R
  Integrator : Integrator  InitialCondition=mot.lamd0
  Integrator1 : Integrator  InitialCondition=mot.lamq0
  MATLAB Function : MATLAB Function  TreatAsAtomicUnit=on
  Product : Product
  Product1 : Product
  Scope : Scope  NumInputPorts=2
  Scope1 : Scope
  Subsystem2 : Subsystem
  Subsystem4 : Subsystem
  Sum : Sum  Inputs=|-+
  lam_d : Outport
  lam_q : Outport  Port=2
  iq : Outport  Port=3
  id : Outport  Port=4
  UA : Outport  Port=5
  UB : Outport  Port=6
  UDQ : Outport  Port=7
  wires:
  thme/1 -> Clarke + Park 2/2(thme)
  Demux1/2 -> Add1/1
  Demux1/1 -> Add/1, MATLAB Function/1(i)
  uabc/1 -> Clarke + Park 2/1(abc), Scope1/1
  [LAM_Q] -> lam_q/1
  [Iq] -> iq/1
  [Id] -> id/1
  [LAM_D] -> lam_d/1
  [LAM_Q] -> 2-D Lookup Table/2
  Gain2/1 -> Add1/3  "R*iq"
  [W_ME] -> Product/1
  [LAM_D] -> Product/2
  w_me/1 -> [W_ME]  "w_me"
  [W_ME] -> Product1/2
  [LAM_D] -> 2-D Lookup Table1/1
  Integrator1/1 -> [LAM_Q], 2-D Lookup Table1/2  "lam_q"
  2-D Lookup Table/1 -> [Id], Scope/1, Gain/1  "id"
  2-D Lookup Table1/1 -> Gain2/1, [Iq], Scope/2  "iq"
  Add1/1 -> Integrator1/1
  Add/1 -> Integrator/1
  [LAM_Q] -> Product1/1
  Integrator/1 -> 2-D Lookup Table/1, [LAM_D]  "lam_d"
  Gain/1 -> Add/3  "R*id"
  Clarke + Park 2/1(dq) -> [U_DQ], Demux1/1
  MATLAB Function/1(y) -> Sum/1
  Clarke + Park 2/3(U_B) -> [U_B]
  Clarke + Park 2/2(U_A) -> [U_A]
  [U_A] -> UA/1
  [U_B] -> UB/1
  Product1/1 -> Add/2
  Product/1 -> Add1/2
  [U_DQ] -> UDQ/1

== system SalientPolePMSM/Synchronous motor1/mechanical system ==
  note: INPUT
  note: OUTPUT
  lam_d : Inport
  lam_q : Inport  Port=2
  iq : Inport  Port=3
  id : Inport  Port=4
  tauL : Inport  Port=5
  Constant : Constant  Value=mot.Tcog
  Demux : Demux  Outputs=2
  Gain : Gain  Gain=3/2*mot.p
  Integrator : Integrator
  Product : Product
  Product1 : Product
  Subtract : Sum  Inputs=+-
  Subtract1 : Sum  Inputs=+--
  Transfer Fcn : TransferFcn  Denominator=[mot.J 0]
  mechanical system : StateSpace  A=[-mot.B/mot.J 0; 1 0]  B=[1/mot.J; 0]  C=eye(2)  D=[0; 0]  InitialCondition=[0, 0]
  thm : Outport
  taum : Outport  Port=2
  wm : Outport  Port=3
  wires:
  lam_q/1 -> Product1/1
  lam_d/1 -> Product/1
  id/1 -> Product1/2
  Gain/1 -> Subtract1/1, taum/1  "taum"
  Product/1 -> Subtract/1
  Product1/1 -> Subtract/2
  tauL/1 -> Subtract1/2
  Subtract/1 -> Gain/1
  iq/1 -> Product/2
  mechanical system/1 -> Demux/1  "wm; thm"
  Constant/1 -> Subtract1/3
  Integrator/1 -> thm/1  "heta_me"
  Subtract1/1 -> mechanical system/1
  Demux/2 -> Integrator/1
  Demux/1 -> wm/1

== system SalientPolePMSM/Synchronous motor2/Subsystem2 ==
  note: INPUTS
  note: OUTPUT
  dq0 : Inport
  thme : Inport  Port=2
  Add2 : Sum  Inputs=+-
  Add3 : Sum
  Cos2 : Trigonometry  Operator=cos
  Demux2 : Demux  Outputs=3
  Gain : Gain  Gain=TAB0_abc  Multiplication=Matrix(K*u) (u vector)
  Mux1 : Mux  Inputs=3
  Product{,1..3} (4 alike) : Product
  Sin2 : Trigonometry
  abc : Outport
  wires:
  dq0/1 -> Demux2/1
  Product/1 -> Add2/1
  Add2/1 -> Mux1/1
  Add3/1 -> Mux1/2
  Product1/1 -> Add2/2
  Cos2/1 -> Product/2, Product3/1
  Demux2/1 -> Product/1, Product2/1
  thme/1 -> Sin2/1, Cos2/1
  Product3/1 -> Add3/2
  Product2/1 -> Add3/1
  Demux2/2 -> Product1/1, Product3/2
  Sin2/1 -> Product2/2, Product1/2
  Mux1/1 -> Gain/1  "AB0"
  Demux2/3 -> Mux1/3
  Gain/1 -> abc/1

== system SalientPolePMSM/Synchronous motor2/electrical equations ==
  note: OUTPUT:
      | dq fluxes
      | dq currents
  note: INPUT VOLTAGES
      | abc AXES and
      | ELECTRICAL
      | SPEED
  uabc : Inport
  thme : Inport  Port=2
  w_me : Inport  Port=3
  2-D Lookup Table : Lookup_n-D  BreakpointsForDimension1=lamdVec  BreakpointsForDimension2=lamqVec  Table=idMap'  InternalRulePriority=Speed  RndMeth=Simplest  InputSameDT=on
      settings: InputPortMap=u0,u1
  2-D Lookup Table1 : Lookup_n-D  BreakpointsForDimension1=lamdVec  BreakpointsForDimension2=lamqVec  Table=iqMap'  InternalRulePriority=Speed  RndMeth=Simplest  InputSameDT=on
      settings: InputPortMap=u0,u1
  Add : Sum  Inputs=++-
  Add1 : Sum  Inputs=+--
  Demux1 : Demux  Outputs=2
  Gain : Gain  Gain=mot.R
  Gain2 : Gain  Gain=mot.R
  Integrator : Integrator  InitialCondition=mot.lamd0
  Integrator1 : Integrator  InitialCondition=mot.lamq0
  Product : Product
  Product1 : Product
  Subsystem1 : Subsystem
  lam_d : Outport
  lam_q : Outport  Port=2
  iq : Outport  Port=3
  id : Outport  Port=4
  wires:
  Gain/1 -> Add/3  "R*id"
  Integrator/1 -> [LAM_D], 2-D Lookup Table/1  "lam_d"
  [LAM_Q] -> Product1/1
  Add/1 -> Integrator/1
  Add1/1 -> Integrator1/1
  2-D Lookup Table1/1 -> [Iq], Gain2/1  "iq"
  2-D Lookup Table/1 -> Gain/1, [Id]  "id"
  Integrator1/1 -> 2-D Lookup Table1/2, [LAM_Q]  "lam_q"
  [LAM_D] -> 2-D Lookup Table1/1
  [W_ME] -> Product1/2
  w_me/1 -> [W_ME]  "w_me"
  [LAM_D] -> Product/2
  [W_ME] -> Product/1
  Gain2/1 -> Add1/3  "R*iq"
  [LAM_Q] -> 2-D Lookup Table/2
  Product/1 -> Add1/2
  Product1/1 -> Add/2
  [LAM_D] -> lam_d/1
  [Id] -> id/1
  [Iq] -> iq/1
  [LAM_Q] -> lam_q/1
  uabc/1 -> Subsystem1/1(abc)
  Demux1/1 -> Add/1
  Demux1/2 -> Add1/1
  thme/1 -> Subsystem1/2(thme)
  Subsystem1/1(dq) -> Demux1/1

== system SalientPolePMSM/Synchronous motor2/mechanical system ==
  note: OUTPUT
  note: INPUT
  lam_d : Inport
  lam_q : Inport  Port=2
  iq : Inport  Port=3
  id : Inport  Port=4
  tauL : Inport  Port=5
  Constant : Constant  Commented=on  Value=mot.Tcog
  Demux : Demux  Outputs=2
  Gain : Gain  Gain=3/2*mot.p
  Product : Product
  Product1 : Product
  Subtract : Sum  Inputs=+-
  Subtract1 : Sum  Inputs=+--
  mechanical system : StateSpace  A=[-mot.B/mot.J 0; 1 0]  B=[1/mot.J; 0]  C=eye(2)  D=[0; 0]  InitialCondition=mot.thm0
  thm : Outport
  taum : Outport  Port=2
  wm : Outport  Port=3
  wires:
  mechanical system/1 -> Demux/1  "wm; thm"
  iq/1 -> Product/2
  Subtract/1 -> Gain/1
  tauL/1 -> Subtract1/2
  Product1/1 -> Subtract/2
  Product/1 -> Subtract/1
  Demux/2 -> thm/1
  Gain/1 -> taum/1, Subtract1/1  "taum"
  Subtract1/1 -> mechanical system/1
  Demux/1 -> wm/1
  id/1 -> Product1/2
  lam_d/1 -> Product/1
  lam_q/1 -> Product1/1

== system SalientPolePMSM/Synchronous motor3/Clarke + Park 1 ==
  note: INPUTS
  note: OUTPUT
  abc : Inport
  thme : Inport  Port=2
  Add2 : Sum
  Add3 : Sum  Inputs=-+
  Cos2 : Trigonometry  Operator=cos
  Demux1 : Demux  Outputs=3
  Demux2 : Demux  Outputs=3
  Gain1 : Gain  Gain=Tabc_AB0  Multiplication=Matrix(K*u) (u vector)
  Gain10 : Gain  Gain=-1/sqrt(3)
  Gain9 : Gain  Gain=2
  Mux1 : Mux  Inputs=2
  Mux2 : Mux  Inputs=3
  Product{,1..3} (4 alike) : Product
  Scope : Scope  NumInputPorts=2
  Sin2 : Trigonometry
  Sum5 : Sum  Inputs=++|
  Terminator : Terminator
  dq : Outport
  wires:
  Demux2/3 -> Terminator/1
  Product/1 -> Add2/1
  Product1/1 -> Add2/2
  Cos2/1 -> Product/2, Product3/1
  Demux2/1 -> Product3/2, Product1/1
  thme/1 -> Cos2/1, Sin2/1
  Product3/1 -> Add3/2
  Product2/1 -> Add3/1
  Demux2/2 -> Product2/1, Product/1
  Sin2/1 -> Product2/2, Product1/2
  Mux1/1 -> dq/1
  Add3/1 -> Mux1/2
  Add2/1 -> Mux1/1
  Sum5/1 -> Gain10/1
  Gain9/1 -> Sum5/2
  Demux1/2 -> Gain9/1
  Demux1/3 -> Mux2/3
  Demux1/1 -> Mux2/1, Sum5/1
  Gain10/1 -> Mux2/2
  abc/1 -> Gain1/1, Demux1/1
  Gain1/1 -> Scope/1, Demux2/1

== system SalientPolePMSM/Synchronous motor3/Rev_Park + Rev_Clarke ==
  note: INPUTS
  dq : Inport
  thme1 : Inport  Port=2
  Add1 : Sum  Inputs=+-
  Add3 : Sum  Inputs=--
  Add4 : Sum
  Cos1 : Trigonometry  Operator=cos
  Demux1 : Demux  Outputs=3
  Gain2 : Gain  Gain=2
  Gain3 : Gain  Gain=-1/sqrt(3)
  Gain4 : Gain  Gain=Talphabeta_abc  Multiplication=Matrix(K*u) (u vector)
  Mux2 : Mux  Inputs=3
  Product{4..7} (4 alike) : Product
  Scope2 : Scope  NumInputPorts=5
  Scope3 : Scope  NumInputPorts=2
  Sin1 : Trigonometry
  Sum1 : Sum  Inputs=++|
  Terminator : Terminator
  abc : Outport
  wires:
  Demux1/3 -> Terminator/1
  dq/1 -> Demux1/1
  Cos1/1 -> Product6/2, Product7/1
  Product5/1 -> Add1/2
  Sin1/1 -> Product5/2, Product4/2
  Product6/1 -> Add4/1
  thme1/1 -> Sin1/1, Cos1/1
  Product4/1 -> Add4/2
  Demux1/1 -> Product5/1, Product6/1
  Product7/1 -> Add1/1
  Demux1/2 -> Product7/2, Product4/1
  Gain3/1 -> Scope2/4, Mux2/2, Add3/2
  Sum1/1 -> Gain3/1
  Gain2/1 -> Sum1/2
  Add3/1 -> Scope2/5, Mux2/3
  Add1/1 -> Scope2/1, Scope2/3, Mux2/1, Add3/1, Sum1/1
  Add4/1 -> Scope2/2, Gain2/1
  ? -> Scope3/2
  Gain4/1 -> Scope3/1
  Mux2/1 -> abc/1

== system SalientPolePMSM/Synchronous motor3/SPM Motor ==
  note: Mechanical Part
  note: Electrical Part
  dq : Inport
  Demux : Demux  Outputs=2
  Divide : Product  Inputs=*/  RndMeth=Zero  SaturateOnIntegerOverflow=on
  Gain : Gain  Gain=mot.Ld
  Gain3 : Gain  Gain=mot.Lq
  Gain4 : Gain  Gain=mot.lammg
  Gain5 : Gain  Gain=3/2*mot.lammg*mot.p
  Gain6 : Gain  Gain=mot.p
  Integrator : Integrator
  MATLAB Function : MATLAB Function  TreatAsAtomicUnit=on
  Product : Product
  Product1 : Product
  Scope : Scope
  Scope2 : Scope
  Scope3 : Scope
  Sum : Sum  Inputs=|++
  Sum1 : Sum  Inputs=-+-
  Sum2 : Sum  Inputs=|+-
  Sum4 : Sum  Inputs=++|
  Transfer Fcn : TransferFcn  Denominator=[mot.Ld mot.R]
  Transfer Fcn1 : TransferFcn  Denominator=[mot.Lq mot.R]
  Transfer Fcn2 : TransferFcn  Denominator=[mot.J mot.B]
  theta_me : Outport
  w_me : Outport  Port=2
  wires:
  dq/1 -> Demux/1
  [TAUL] -> Sum2/2
  Sum/1 -> Transfer Fcn/1
  Gain3/1 -> Sum/2
  Gain/1 -> Sum1/1
  Integrator/1 -> Sum4/2  "theta_me"
  Sum2/1 -> Transfer Fcn2/1
  Transfer Fcn/1 -> Product/1  "id"
  Gain6/1 -> Product/2, Product1/1, Integrator/1, w_me/1, Scope3/1, Gain4/1  "w_me"
  Product/1 -> Gain/1
  Demux/2 -> Sum1/2
  Product1/1 -> Gain3/1
  Gain4/1 -> Sum1/3
  Sum1/1 -> Transfer Fcn1/1
  Sum4/1 -> theta_me/1
  Demux/1 -> Sum/1
  Transfer Fcn1/1 -> Gain5/1, Scope2/1, Product1/2  "iq"
  Transfer Fcn2/1 -> Gain6/1  "w_m"
  MATLAB Function/1(B) -> Divide/2
  Gain5/1 -> Sum2/1, Scope/1  "tau"

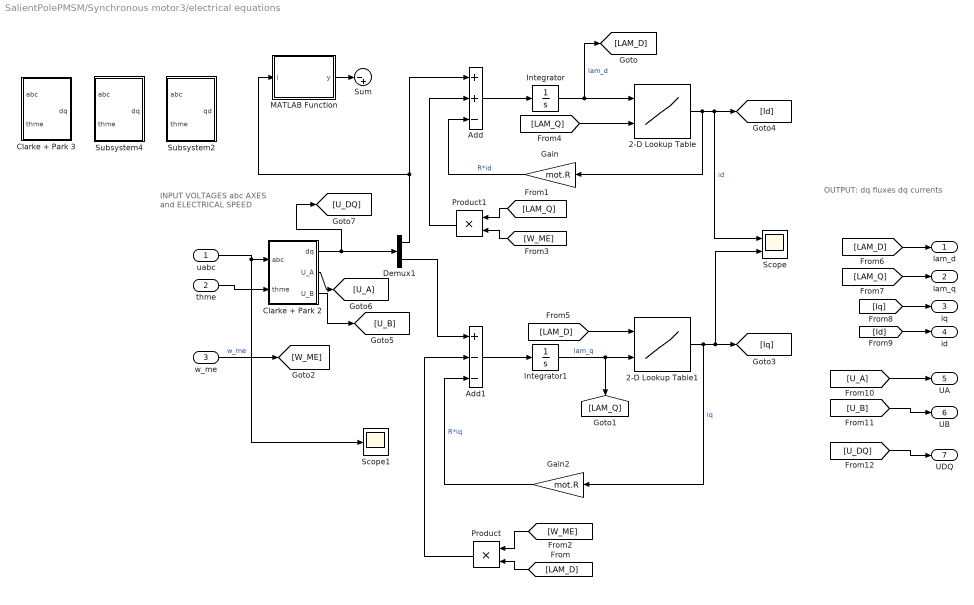
== system SalientPolePMSM/Synchronous motor3/electrical equations ==
  note: INPUT VOLTAGES
      | abc AXES and
      | ELECTRICAL
      | SPEED
  note: OUTPUT:
      | dq fluxes
      | dq currents
  uabc : Inport
  thme : Inport  Port=2
  w_me : Inport  Port=3
  2-D Lookup Table : Lookup_n-D  BreakpointsForDimension1=lamdVec  BreakpointsForDimension2=lamqVec  Table=idMap'  InternalRulePriority=Speed  RndMeth=Simplest  InputSameDT=on
      settings: InputPortMap=u0,u1
  2-D Lookup Table1 : Lookup_n-D  BreakpointsForDimension1=lamdVec  BreakpointsForDimension2=lamqVec  Table=iqMap'  InternalRulePriority=Speed  RndMeth=Simplest  InputSameDT=on
      settings: InputPortMap=u0,u1
  Add : Sum  Inputs=++-
  Add1 : Sum  Inputs=+--
  Clarke + Park 2 : Subsystem
  Clarke + Park 3 : Subsystem
  Demux1 : Demux  Outputs=2
  Gain : Gain  Gain=mot.R
  Gain2 : Gain  Gain=mot.R
  Integrator : Integrator  InitialCondition=mot.lamd0
  Integrator1 : Integrator  InitialCondition=mot.lamq0
  MATLAB Function : MATLAB Function  TreatAsAtomicUnit=on
  Product : Product
  Product1 : Product
  Scope : Scope  NumInputPorts=2
  Scope1 : Scope
  Subsystem2 : Subsystem
  Subsystem4 : Subsystem
  Sum : Sum  Inputs=|-+
  lam_d : Outport
  lam_q : Outport  Port=2
  iq : Outport  Port=3
  id : Outport  Port=4
  UA : Outport  Port=5
  UB : Outport  Port=6
  UDQ : Outport  Port=7
  wires:
  thme/1 -> Clarke + Park 2/2(thme)
  Demux1/2 -> Add1/1
  Demux1/1 -> Add/1, MATLAB Function/1(i)
  uabc/1 -> Clarke + Park 2/1(abc), Scope1/1
  [LAM_Q] -> lam_q/1
  [Iq] -> iq/1
  [Id] -> id/1
  [LAM_D] -> lam_d/1
  [LAM_Q] -> 2-D Lookup Table/2
  Gain2/1 -> Add1/3  "R*iq"
  [W_ME] -> Product/1
  [LAM_D] -> Product/2
  w_me/1 -> [W_ME]  "w_me"
  [W_ME] -> Product1/2
  [LAM_D] -> 2-D Lookup Table1/1
  Integrator1/1 -> [LAM_Q], 2-D Lookup Table1/2  "lam_q"
  2-D Lookup Table/1 -> [Id], Scope/1, Gain/1  "id"
  2-D Lookup Table1/1 -> Gain2/1, [Iq], Scope/2  "iq"
  Add1/1 -> Integrator1/1
  Add/1 -> Integrator/1
  [LAM_Q] -> Product1/1
  Integrator/1 -> 2-D Lookup Table/1, [LAM_D]  "lam_d"
  Gain/1 -> Add/3  "R*id"
  Clarke + Park 2/1(dq) -> [U_DQ], Demux1/1
  MATLAB Function/1(y) -> Sum/1
  Clarke + Park 2/3(U_B) -> [U_B]
  Clarke + Park 2/2(U_A) -> [U_A]
  [U_A] -> UA/1
  [U_B] -> UB/1
  Product1/1 -> Add/2
  Product/1 -> Add1/2
  [U_DQ] -> UDQ/1

== system SalientPolePMSM/Synchronous motor3/mechanical system ==
  note: INPUT
  note: OUTPUT
  lam_d : Inport
  lam_q : Inport  Port=2
  iq : Inport  Port=3
  id : Inport  Port=4
  tauL : Inport  Port=5
  Constant : Constant  Value=mot.Tcog
  Demux : Demux  Outputs=2
  Gain : Gain  Gain=3/2*mot.p
  Product : Product
  Product1 : Product
  Subtract : Sum  Inputs=+-
  Subtract1 : Sum  Inputs=+--
  Transfer Fcn : TransferFcn  Denominator=[mot.J 0]
  mechanical system : StateSpace  A=[-mot.B/mot.J 0; 1 0]  B=[1/mot.J; 0]  C=eye(2)  D=[0; 0]  InitialCondition=[0, 0]
  thm : Outport
  taum : Outport  Port=2
  wm : Outport  Port=3
  wires:
  lam_q/1 -> Product1/1
  lam_d/1 -> Product/1
  id/1 -> Product1/2
  Gain/1 -> Subtract1/1, taum/1  "taum"
  Product/1 -> Subtract/1
  Product1/1 -> Subtract/2
  tauL/1 -> Subtract1/2
  Subtract/1 -> Gain/1
  iq/1 -> Product/2
  mechanical system/1 -> Demux/1  "wm; thm"
  Constant/1 -> Subtract1/3
  Demux/2 -> thm/1  "theta_me"
  Subtract1/1 -> mechanical system/1
  Demux/1 -> wm/1

== system SalientPolePMSM/DT SENSORLESS ALGORITHM AB/Normalized and improved PLL2/Discrete PI ==
  e : Inport
  Delay : Delay  DelayLength=1
  Gain6 : Gain  Gain=Obs.PI.ki*Obs.Ts*0.0001
  Gain7 : Gain  Gain=Obs.PI.kp*0.000002
  Sum2 : Sum  Inputs=++|
  Sum3 : Sum  Inputs=++|
  w_est : Outport
  wires:
  Sum3/1 -> w_est/1  "w_est"
  Gain6/1 -> Sum3/1
  Sum2/1 -> Delay/1
  Delay/1 -> Sum2/1, Gain6/1
  e/1 -> Sum2/2, Gain7/1
  Gain7/1 -> Sum3/2

== system SalientPolePMSM/DT SENSORLESS ALGORITHM DQ/Normalized and improved PLL3/Discrete PI ==
  e : Inport
  Delay : Delay  DelayLength=1
  Gain6 : Gain  Gain=Obs.PI.ki*Obs.Ts*70
  Gain7 : Gain  Gain=Obs.PI.kp*5
  Sum2 : Sum  Inputs=++|
  Sum3 : Sum  Inputs=++|
  w_est : Outport
  wires:
  Sum3/1 -> w_est/1  "w_est"
  Gain6/1 -> Sum3/1
  Sum2/1 -> Delay/1
  Delay/1 -> Sum2/1, Gain6/1
  e/1 -> Sum2/2, Gain7/1
  Gain7/1 -> Sum3/2

== system SalientPolePMSM/FOC1/Changed1/Subsystem ==
  A : Inport
  B : Inport  Port=2
  Gain2 : Gain  Gain=2
  Gain3 : Gain  Gain=-1/sqrt(3)
  Product5 : Product
  d : Outport
  q : Outport  Port=2
  wires:
  B/1 -> Gain2/1
  A/1 -> d/1, Product5/1
  Gain3/1 -> q/1
  Gain2/1 -> Product5/2
  Product5/1 -> Gain3/1

== system SalientPolePMSM/FOC1/INVERTER1/INVERTER power driver ==
  note: INVERTER:
      | (-Ubus/2  :  +Ubus/2)
  note: INPUTS:
  note: OUTPUTS:
  note: solo Tpwm/2 perchè
      | controllo tempo discreto
  duties : Inport
  uBus : Inport  Port=2
  iabc : Inport  Port=3
  Constant1 : Constant  Value=0.5
  Inverter non idealities : Subsystem
  Product : Product
  Subtract : Sum  Inputs=+-
  Transport Delay : TransportDelay  DelayTime=inv.Tpwm/2
  delay_aproximation : Subsystem  Commented=on
  uabc_n* : Outport
  uabc_n*nonideal : Outport  Port=2
  wires:
  Transport Delay/1 -> uabc_n*/1
  iabc/1 -> Inverter non idealities/3(iabc)
  duties/1 -> Subtract/1
  Inverter non idealities/1(uabc_dist) -> uabc_n*nonideal/1
  Constant1/1 -> Subtract/2
  uBus/1 -> Inverter non idealities/2(uBus), Product/2
  Product/1 -> Transport Delay/1, Inverter non idealities/1(uabc)  "uabc"
  Subtract/1 -> Product/1

== system SalientPolePMSM/FOC1/INVERTER1/SVM algorithm ==
  note: INPUTS:
      | voltage references
      | Alpha Beta axes
  note: Decide whether
      | to use circle or
      | hexagonal saturation
  note: OUTPUT
  UABref : Inport  PortDimensions=2
  uBus : Inport  Port=2  PortDimensions=1
  MATLAB Function : MATLAB Function  TreatAsAtomicUnit=on
  MATLAB Function1 : MATLAB Function  TreatAsAtomicUnit=on
  MATLAB Function2 : MATLAB Function  TreatAsAtomicUnit=on
  MATLAB Function3 : MATLAB Function  TreatAsAtomicUnit=on
  Manual Switch : ManualSwitch  CurrentSetting=0
  OR : Logic  Operator=OR  IconShape=distinctive  AllPortsSameDT=off  OutDataTypeStr=boolean
  XY Graph : simulink/Sinks/XY Graph  xmin=-350  xmax=350  ymin=-350  ymax=350  st=-1
  duties : Outport  PortDimensions=3
  satON : Outport  Port=2  PortDimensions=1
  wires:
  OR/1 -> satON/1
  MATLAB Function1/2(satON) -> OR/2
  MATLAB Function3/4(satON) -> OR/1
  MATLAB Function3/3(duties) -> duties/1
  uBus/1 -> [UBUS]
  Manual Switch/1 -> MATLAB Function2/2(uABref), MATLAB Function3/3(uABref)
  MATLAB Function1/1(uABref_sat) -> Manual Switch/2
  [UBUS] -> MATLAB Function1/2(uBus)
  MATLAB Function2/1(Tm_m1_0) -> MATLAB Function3/2(Tm_m1_0)
  UABref/1 -> MATLAB Function/1(uABref), Manual Switch/1, MATLAB Function1/1(UABref)
  [UBUS] -> MATLAB Function2/3(uBus)
  MATLAB Function/1(sector) -> MATLAB Function2/1(sid), MATLAB Function3/1(sid)
  MATLAB Function3/2(uBref_sat) -> XY Graph/2  "uBref_sat"
  MATLAB Function3/1(uAref_sat) -> XY Graph/1  "uAref_sat"

== system SalientPolePMSM/FOC1/INVERTER2/INVERTER power driver ==
  note: INVERTER:
      | (-Ubus/2  :  +Ubus/2)
  note: INPUTS:
  note: OUTPUTS:
  note: solo Tpwm/2 perchè
      | controllo tempo discreto
  duties : Inport
  uBus : Inport  Port=2
  iabc : Inport  Port=3
  Constant1 : Constant  Value=0.5
  Inverter non idealities : Subsystem  Commented=on
  Product : Product
  Subtract : Sum  Inputs=+-
  Transport Delay : TransportDelay  DelayTime=inv.Tpwm/2
  delay_aproximation : Subsystem  Commented=on
  uabc_n* : Outport
  uabc_n*nonideal : Outport  Port=2
  wires:
  iabc/1 -> Inverter non idealities/3(iabc)
  duties/1 -> Subtract/1
  Inverter non idealities/1(uabc_dist) -> uabc_n*nonideal/1
  Constant1/1 -> Subtract/2
  uBus/1 -> Inverter non idealities/2(uBus), Product/2
  Product/1 -> Inverter non idealities/1(uabc), Transport Delay/1  "uabc"
  Subtract/1 -> Product/1
  Transport Delay/1 -> uabc_n*/1

== system SalientPolePMSM/FOC1/INVERTER2/SVM algorithm ==
  note: INPUTS:
      | voltage references
      | Alpha Beta axes
  note: OUTPUT
  VABref : Inport  PortDimensions=2
  uBus : Inport  Port=2  PortDimensions=1
  Gain : Gain  Gain=1000
  MATLAB Function : MATLAB Function  Commented=on  TreatAsAtomicUnit=on  SystemSampleTime=inv.Ts
  MATLAB Function1 : MATLAB Function  TreatAsAtomicUnit=on  SystemSampleTime=inv.Ts
  MATLAB Function2 : MATLAB Function  TreatAsAtomicUnit=on  SystemSampleTime=inv.Ts
  MATLAB Function4 : MATLAB Function  Commented=on  TreatAsAtomicUnit=on  SystemSampleTime=inv.Ts
  Mux : Mux  Commented=on  Inputs=3
  Mux1 : Mux  Inputs=3
  Scope : Scope  Commented=on  NumInputPorts=3
  Scope1 : Scope  Commented=on  NumInputPorts=2
  Scope2 : Scope  NumInputPorts=2
  duties : Outport  PortDimensions=3
  wires:
  Mux/1 -> MATLAB Function/1(XYZ)
  MATLAB Function4/3(Z) -> Scope/3, Mux/3
  MATLAB Function4/2(Y) -> Scope/2, Mux/2
  MATLAB Function4/1(X) -> Scope/1, Mux/1
  MATLAB Function/2(duty) -> Scope1/1
  uBus/1 -> [UBUS]
  VABref/1 -> MATLAB Function4/1(VABref), Gain/1
  MATLAB Function/1(sector) -> Scope1/2
  MATLAB Function1/3(Z) -> Mux1/3
  MATLAB Function1/2(Y) -> Mux1/2
  MATLAB Function1/1(X) -> Mux1/1
  Gain/1 -> MATLAB Function1/1(VABref)
  Mux1/1 -> MATLAB Function2/1(XYZ)
  MATLAB Function2/2(duty) -> duties/1, Scope2/1
  MATLAB Function2/1(sector) -> Scope2/2

== system SalientPolePMSM/FOC2/Changed1/Subsystem ==
  A : Inport
  B : Inport  Port=2
  Gain2 : Gain  Gain=2
  Gain3 : Gain  Gain=-1/sqrt(3)
  Product5 : Product
  d : Outport
  q : Outport  Port=2
  wires:
  B/1 -> Gain2/1
  A/1 -> d/1, Product5/1
  Gain3/1 -> q/1
  Gain2/1 -> Product5/2
  Product5/1 -> Gain3/1

== system SalientPolePMSM/FOC2/INVERTER1/INVERTER power driver ==
  note: INVERTER:
      | (-Ubus/2  :  +Ubus/2)
  note: INPUTS:
  note: OUTPUTS:
  note: solo Tpwm/2 perchè
      | controllo tempo discreto
  duties : Inport
  uBus : Inport  Port=2
  iabc : Inport  Port=3
  Constant1 : Constant  Value=0.5
  Inverter non idealities : Subsystem
  Product : Product
  Subtract : Sum  Inputs=+-
  Transport Delay : TransportDelay  DelayTime=inv.Tpwm/2
  delay_aproximation : Subsystem  Commented=on
  uabc_n* : Outport
  uabc_n*nonideal : Outport  Port=2
  wires:
  Transport Delay/1 -> uabc_n*/1
  iabc/1 -> Inverter non idealities/3(iabc)
  duties/1 -> Subtract/1
  Inverter non idealities/1(uabc_dist) -> uabc_n*nonideal/1
  Constant1/1 -> Subtract/2
  uBus/1 -> Inverter non idealities/2(uBus), Product/2
  Product/1 -> Transport Delay/1, Inverter non idealities/1(uabc)  "uabc"
  Subtract/1 -> Product/1

== system SalientPolePMSM/FOC2/INVERTER1/SVM algorithm ==
  note: INPUTS:
      | voltage references
      | Alpha Beta axes
  note: Decide whether
      | to use circle or
      | hexagonal saturation
  note: OUTPUT
  UABref : Inport  PortDimensions=2
  uBus : Inport  Port=2  PortDimensions=1
  MATLAB Function : MATLAB Function  TreatAsAtomicUnit=on
  MATLAB Function1 : MATLAB Function  TreatAsAtomicUnit=on
  MATLAB Function2 : MATLAB Function  TreatAsAtomicUnit=on
  MATLAB Function3 : MATLAB Function  TreatAsAtomicUnit=on
  Manual Switch : ManualSwitch  CurrentSetting=0
  OR : Logic  Operator=OR  IconShape=distinctive  AllPortsSameDT=off  OutDataTypeStr=boolean
  XY Graph : simulink/Sinks/XY Graph  xmin=-350  xmax=350  ymin=-350  ymax=350  st=-1
  duties : Outport  PortDimensions=3
  satON : Outport  Port=2  PortDimensions=1
  wires:
  OR/1 -> satON/1
  MATLAB Function1/2(satON) -> OR/2
  MATLAB Function3/4(satON) -> OR/1
  MATLAB Function3/3(duties) -> duties/1
  uBus/1 -> [UBUS]
  Manual Switch/1 -> MATLAB Function2/2(uABref), MATLAB Function3/3(uABref)
  MATLAB Function1/1(uABref_sat) -> Manual Switch/2
  [UBUS] -> MATLAB Function1/2(uBus)
  MATLAB Function2/1(Tm_m1_0) -> MATLAB Function3/2(Tm_m1_0)
  UABref/1 -> MATLAB Function/1(uABref), Manual Switch/1, MATLAB Function1/1(UABref)
  [UBUS] -> MATLAB Function2/3(uBus)
  MATLAB Function/1(sector) -> MATLAB Function2/1(sid), MATLAB Function3/1(sid)
  MATLAB Function3/2(uBref_sat) -> XY Graph/2  "uBref_sat"
  MATLAB Function3/1(uAref_sat) -> XY Graph/1  "uAref_sat"
